simulink model "Punktmodell"  (R2024a)
settings: Solver=VariableStepAuto  StartTime=0.0  StopTime=10.0  RelTol=1e-3
model workspace (MAT data in the model file):
  g = 9.81
  m = 530
  m_L = Simulink.Parameter
  m_L.Value = 0.52
  m_L.Complexity = 'real'
  m_L.Dimensions = [1 1]
  m_L.DataType = 'auto'
  m_L.DocUnits = 'kg'
  m_R = Simulink.Parameter
  m_R.Value = 0.01
  m_R.Complexity = 'real'
  m_R.Dimensions = [1 1]
  m_R.DataType = 'auto'
  m_R.DocUnits = 'kg'
  mue = 0.002
  r = 0.01
settings Model: Creator=jakob  LastModifiedBy=jakob

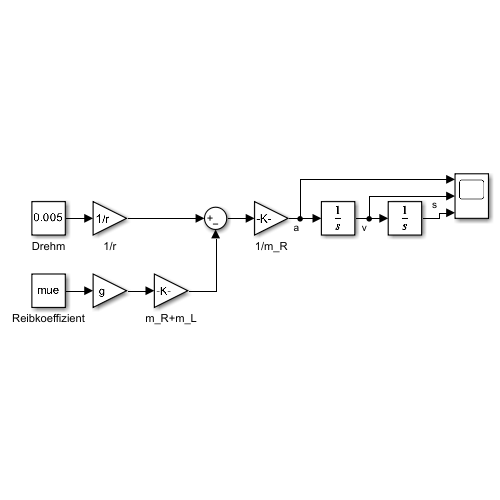
[thumbnail: Simulink's stored preview of the top-level diagram]
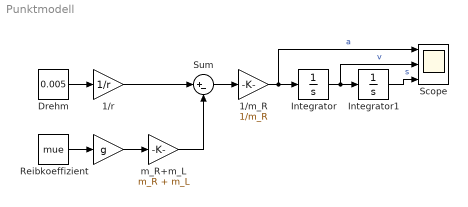
== system Punktmodell ==
  " " : Gain  Gain=g
  1/m_R : Gain  Gain=1/m_R
  1/r : Gain  Gain=1/r
  Drehm : Constant  Value=0.005
  Integrator : Integrator  InitialCondition=1
  Integrator1 : Integrator
  Reibkoeffizient : Constant  Value=mue
  Scope : Scope  NumInputPorts=3
  Sum : Sum  Inputs=|+-
  m_R+m_L : Gain  Gain=m_R + m_L
  wires:
  Reibkoeffizient/1 -> " "/1
  Integrator1/1 -> Scope/3  "s"
  Integrator/1 -> Scope/2, Integrator1/1  "v"
  1/r/1 -> Sum/1
  Drehm/1 -> 1/r/1
  " "/1 -> m_R+m_L/1
  m_R+m_L/1 -> Sum/2
  Sum/1 -> 1/m_R/1
  1/m_R/1 -> Scope/1, Integrator/1  "a"
